simulink model "thruster_controller"  (Simulink 6.0)
settings: Solver=ode45  StartTime=0.0  StopTime=100  RelTol=1e-3
libraries: rov_design_analysis x1, simulink_extras x1
settings Model: LastModifiedBy=c chin

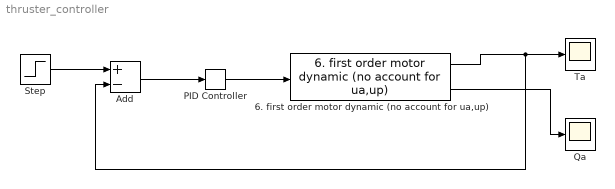
== system thruster_controller ==
  6. first order motor dynamic (no account for ua,up) : rov_design_analysis/Propeller Models/6. first order motor dynamic (no account for ua,up)
  Add : Sum  Inputs=+-  OutScaling=2^-10
  "PID Controller " : simulink_extras/Additional Linear/PID Controller  P=11  I=0  D=11
  Qa : Scope
  Step : Step  After=10  SampleTime=0
  Ta : Scope
  wires:
  "PID Controller "/1 -> 6. first order motor dynamic (no account for ua,up)/1
  Add/1 -> "PID Controller "/1
  Step/1 -> Add/1
  6. first order motor dynamic (no account for ua,up)/1 -> Ta/1, Add/2
  6. first order motor dynamic (no account for ua,up)/2 -> Qa/1
